simulink model "newtons_cradle"  (R2013b)
settings: Solver=ode45  StartTime=0.0  StopTime=10.0  RelTol=1e-3
settings Model: Creator=Daniel  LastModifiedBy=Daniel

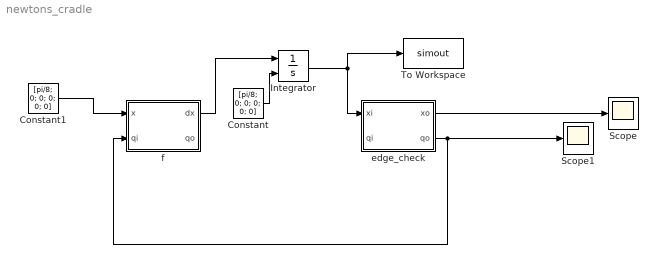
== system newtons_cradle ==
  Constant : Constant  Value=[pi/8; 0; 0; 0; 0; 0]
  Constant1 : Constant  Value=[pi/8; 0; 0; 0; 0; 0]
  Integrator : Integrator  InitialConditionSource=external
  Scope : Scope
  Scope1 : Scope
  To Workspace : ToWorkspace  VariableName=simout  SampleTime=-1  SaveFormat=Timeseries
  edge_check : MATLAB Function  TreatAsAtomicUnit=on
  f : MATLAB Function  TreatAsAtomicUnit=on
  wires:
  f/1(dx) -> Integrator/1
  Integrator/1 -> edge_check/1(xi), To Workspace/1
  ? -> edge_check/2(qi)
  edge_check/1(xo) -> Scope/1
  edge_check/2(qo) -> Scope1/1, f/2(qi)
  Constant/1 -> Integrator/2
  Constant1/1 -> f/1(x)

== matlab function newtons_cradle/edge_check ==
  data: xi input; xo output; qi input; qo output
function [xo , qo] = e(xi, qi)
%#codegen
xo = xi; %pre-assignment
qo = qi; %pre-assignment

switch qi
    case 1
        x_in_guard12 = ( xi(1) <= 0 ) && ( xi(2) < 0 );
        
        if x_in_guard12
            qo = 2;
            xo(1) = 0;
            xo(2) = 0;
            xo(3) = 0;
            xo(4) = xi(2);
            xo(5) = 0;
            xo(6) = 0;
        else
            
        end
    case 2
        x_in_guard21 = ( xi(3) ~= 0 ) && ( xi(4) > 0 ) ;
        x_in_guard23 = ( xi(3) ~= 0 ) && ( xi(4) < 0 ) ;
        
        if x_in_guard21
            qo = 1;
            xo(1) = 0;
            xo(2) = xi(4);
            xo(3) = 0;
            xo(4) = 0;
            xo(5) = 0;
            xo(6) = 0;
        end
        if x_in_guard23
            qo = 3;
            xo(1) = 0;
            xo(2) = 0;
            xo(3) = 0;
            xo(4) = 0;
            xo(5) = 0;
            xo(6) = xi(4);
        end
        
    case 3
        x_in_guard32 = ( xi(5) >= 0 ) && ( xi(6) > 0 ) ;
        
        if x_in_guard32
            qo = 2;
            xo(1) = 0;
            xo(2) = 0;
            xo(3) = 0;
            xo(4) = xi(6);
            xo(5) = 0;
            xo(6) = 0;
        end
        
    otherwise
        error = 'qi out of bounds in edge_check function'
end

end

== matlab function newtons_cradle/f ==
  data: x input; dx output; qi input; qo output
function [dx, qo] = f(x, qi)
%#codegen
%global g;
%global l;
g = 9.81;
l = 10;

dx = zeros(size(x));            %pre-allocation

switch qi
    case 1
        dx = [x(2)             ; %theta1'
              -(g/l)*sin(x(1)) ; %omega1'
              x(4)             ; %theta2'
              0                ; %omega2'
              x(6)             ; %theta3'
              0                ];%omega3'
    case 2
        dx = [x(2)             ; %theta1'
              0                ; %omega1'
              x(4)             ; %theta2'
              -(g/l)*sin(x(3)) ; %omega2'
              x(6)             ; %theta3'
              0                ];%omega3'
    case 3
        dx = [x(2)             ; %theta1'
              0                ; %omega1'
              x(4)             ; %theta2'
              0                ; %omega2'
              x(6)             ; %theta3'
              -(g/l)*sin(x(5)) ];%omega3'
    otherwise
        error = 'qi out of bounds in f function'
end

qo = qi;
end
